simulink model "VehCtrlMdel240818"  (R2018b)
settings: Solver=FixedStepDiscrete  StartTime=0.0  StopTime=10.0  FixedStep=0.0005  RelTol=1e-3  EnableMultiTasking=on
values from neighbouring files (symbols this model uses):
  Ax_OffSet = 0.0    [VehCtrlMdelDictionary.sldd]
  Ay_OffSet = 0.0    [VehCtrlMdelDictionary.sldd]
  Caf = 460.0    [VehCtrlMdelDictionary.sldd]    (also in trqvparameter.m = 460)
  Car = 440.0    [VehCtrlMdelDictionary.sldd]    (also in trqvparameter.m = 440)
  dwf = 1.2    [VehCtrlMdelDictionary.sldd]    (also in trqvparameter.m)
  Iz = 105.0    [VehCtrlMdelDictionary.sldd]    (also in trqvparameter.m = 105)
  Ki = 1.0    [VehCtrlMdelDictionary.sldd]    (also in trqvparameter.m = 20)
  Kp = 2.0    [VehCtrlMdelDictionary.sldd]    (also in trqvparameter.m = 30)
  Ldwf = 1.2    [VehCtrlMdelDictionary.sldd]    (also in trqvparameter.m)
  Ldwr = 1.16    [VehCtrlMdelDictionary.sldd]    (also in trqvparameter.m)
  lf = 0.761    [VehCtrlMdelDictionary.sldd]    (also in trqvparameter.m)
  lr = 0.831    [VehCtrlMdelDictionary.sldd]    (also in trqvparameter.m)
  m = 340.0    [VehCtrlMdelDictionary.sldd]    (also in trqvparameter.m = 340)
  Offset_Angle = 0.0    [VehCtrlMdelDictionary.sldd]
  Qa = 0.1    [VehCtrlMdelDictionary.sldd]    (also in trqvparameter.m)
  Ra = 2.0    [VehCtrlMdelDictionary.sldd]    (also in trqvparameter.m = 2)
  RearRatio = 0.8    [VehCtrlMdelDictionary.sldd]
  Rt = 0.2    [VehCtrlMdelDictionary.sldd]    (also in trqvparameter.m)
  thr1 = 2.0    [VehCtrlMdelDictionary.sldd]    (also in trqvparameter.m = 2)
  thr2 = 0.5    [VehCtrlMdelDictionary.sldd]    (also in trqvparameter.m)
  thr3 = 0.8    [VehCtrlMdelDictionary.sldd]    (also in trqvparameter.m)
  thr4 = 0.5    [VehCtrlMdelDictionary.sldd]    (also in trqvparameter.m)
  thr5 = -0.5    [VehCtrlMdelDictionary.sldd]    (also in trqvparameter.m)
  TrqRquRate = 0.1    [VehCtrlMdelDictionary.sldd]    (also in trqvparameter.m)
  YawRate_OffSet = 0.0    [VehCtrlMdelDictionary.sldd]
undefined symbols (not defined in the file or in its folder): DiscIntNeverNeededParam, I_AN07_5V, I_AN08_5V, I_AN10_5V, I_SW01_L, I_SW02_L, I_SW03_L, O_SW12_HS1A, O_SW14_HS1A, PWM3
libraries: simulink x126, ec5744lib x77, canmsglib x18
(part 5 of 5)

== system VehCtrlMdel240818/Input_Processing/Subsystem/WhlSlpageJudgment/加速度差判断/Filter1 ==
  In : Inport
  Add : Sum
  Constant : Constant  Value=single(-100)
  Constant1 : Constant  Value=single(100)
  Constant2 : Constant  Value=single(100)
  Constant3 : Constant  Value=single(-100)
  Gain : Gain  Gain=0.3
  Gain1 : Gain  Gain=0.7
  Rate Limiter Dynamic : simulink/Discontinuities/Rate Limiter Dynamic
      settings: SourceProductName=Simulink
  Saturation Dynamic : simulink/Discontinuities/Saturation Dynamic  OutMin=[]  OutMax=[]  OutDataTypeStr=Inherit: Same as second input  OutDataType=fixdt(1, 16)  OutScaling=2^-10  DoSatur=off
  Unit Delay : UnitDelay  SampleTime=-1
  Out : Outport  VectorParamsAs1DForOutWhenUnconnected=on
  wires:
  Rate Limiter Dynamic/1 -> Unit Delay/1, Gain1/1
  Gain1/1 -> Add/2
  Add/1 -> Out/1
  Gain/1 -> Add/1
  Unit Delay/1 -> Gain/1
  Constant3/1 -> Rate Limiter Dynamic/3
  Constant2/1 -> Rate Limiter Dynamic/1
  Constant/1 -> Saturation Dynamic/3
  Constant1/1 -> Saturation Dynamic/1
  Saturation Dynamic/1 -> Rate Limiter Dynamic/2
  In/1 -> Saturation Dynamic/2

== system VehCtrlMdel240818/Input_Processing/Subsystem/WhlSlpageJudgment/加速度差判断/Filter2 ==
  In : Inport
  Add : Sum
  Constant : Constant  Value=single(-100)
  Constant1 : Constant  Value=single(100)
  Constant2 : Constant  Value=single(100)
  Constant3 : Constant  Value=single(-100)
  Gain : Gain  Gain=0.3
  Gain1 : Gain  Gain=0.7
  Rate Limiter Dynamic : simulink/Discontinuities/Rate Limiter Dynamic
      settings: SourceProductName=Simulink
  Saturation Dynamic : simulink/Discontinuities/Saturation Dynamic  OutMin=[]  OutMax=[]  OutDataTypeStr=Inherit: Same as second input  OutDataType=fixdt(1, 16)  OutScaling=2^-10  DoSatur=off
  Unit Delay : UnitDelay  SampleTime=-1
  Out : Outport  VectorParamsAs1DForOutWhenUnconnected=on
  wires:
  In/1 -> Saturation Dynamic/2
  Saturation Dynamic/1 -> Rate Limiter Dynamic/2
  Constant1/1 -> Saturation Dynamic/1
  Constant/1 -> Saturation Dynamic/3
  Constant2/1 -> Rate Limiter Dynamic/1
  Constant3/1 -> Rate Limiter Dynamic/3
  Unit Delay/1 -> Gain/1
  Gain/1 -> Add/1
  Add/1 -> Out/1
  Gain1/1 -> Add/2
  Rate Limiter Dynamic/1 -> Gain1/1, Unit Delay/1

== system VehCtrlMdel240818/Input_Processing/Subsystem/WhlSlpageJudgment/加速度差判断/Filter3 ==
  In : Inport
  Add : Sum
  Constant : Constant  Value=single(-100)
  Constant1 : Constant  Value=single(100)
  Constant2 : Constant  Value=single(100)
  Constant3 : Constant  Value=single(-100)
  Gain : Gain  Gain=0.3
  Gain1 : Gain  Gain=0.7
  Rate Limiter Dynamic : simulink/Discontinuities/Rate Limiter Dynamic
      settings: SourceProductName=Simulink
  Saturation Dynamic : simulink/Discontinuities/Saturation Dynamic  OutMin=[]  OutMax=[]  OutDataTypeStr=Inherit: Same as second input  OutDataType=fixdt(1, 16)  OutScaling=2^-10  DoSatur=off
  Unit Delay : UnitDelay  SampleTime=-1
  Out : Outport  VectorParamsAs1DForOutWhenUnconnected=on
  wires:
  Rate Limiter Dynamic/1 -> Unit Delay/1, Gain1/1
  Gain1/1 -> Add/2
  Add/1 -> Out/1
  Gain/1 -> Add/1
  Unit Delay/1 -> Gain/1
  Constant3/1 -> Rate Limiter Dynamic/3
  Constant2/1 -> Rate Limiter Dynamic/1
  Constant/1 -> Saturation Dynamic/3
  Constant1/1 -> Saturation Dynamic/1
  Saturation Dynamic/1 -> Rate Limiter Dynamic/2
  In/1 -> Saturation Dynamic/2

== system VehCtrlMdel240818/Input_Processing/Subsystem/WhlSlpageJudgment/加速度差的微分的判断/Filter ==
  In : Inport
  Add : Sum
  Constant : Constant  Value=single(-100)
  Constant1 : Constant  Value=single(100)
  Constant2 : Constant  Value=single(20)
  Constant3 : Constant  Value=single(-20)
  Gain : Gain  Gain=0.5
  Gain1 : Gain  Gain=0.5
  Rate Limiter Dynamic : simulink/Discontinuities/Rate Limiter Dynamic
      settings: SourceProductName=Simulink
  Saturation Dynamic : simulink/Discontinuities/Saturation Dynamic  OutMin=[]  OutMax=[]  OutDataTypeStr=Inherit: Same as second input  OutDataType=fixdt(1, 16)  OutScaling=2^-10  DoSatur=off
  Unit Delay : UnitDelay  SampleTime=-1
  Out : Outport  VectorParamsAs1DForOutWhenUnconnected=on
  wires:
  In/1 -> Saturation Dynamic/2
  Saturation Dynamic/1 -> Rate Limiter Dynamic/2
  Constant1/1 -> Saturation Dynamic/1
  Constant/1 -> Saturation Dynamic/3
  Constant2/1 -> Rate Limiter Dynamic/1
  Constant3/1 -> Rate Limiter Dynamic/3
  Unit Delay/1 -> Gain/1
  Gain/1 -> Add/1
  Add/1 -> Out/1
  Gain1/1 -> Add/2
  Rate Limiter Dynamic/1 -> Gain1/1, Unit Delay/1

== system VehCtrlMdel240818/Input_Processing/Subsystem/WhlSlpageJudgment/加速度差的微分的判断/Filter1 ==
  In : Inport
  Add : Sum
  Constant : Constant  Value=single(-100)
  Constant1 : Constant  Value=single(100)
  Constant2 : Constant  Value=single(20)
  Constant3 : Constant  Value=single(-20)
  Gain : Gain  Gain=0.5
  Gain1 : Gain  Gain=0.5
  Rate Limiter Dynamic : simulink/Discontinuities/Rate Limiter Dynamic
      settings: SourceProductName=Simulink
  Saturation Dynamic : simulink/Discontinuities/Saturation Dynamic  OutMin=[]  OutMax=[]  OutDataTypeStr=Inherit: Same as second input  OutDataType=fixdt(1, 16)  OutScaling=2^-10  DoSatur=off
  Unit Delay : UnitDelay  SampleTime=-1
  Out : Outport  VectorParamsAs1DForOutWhenUnconnected=on
  wires:
  Rate Limiter Dynamic/1 -> Unit Delay/1, Gain1/1
  Gain1/1 -> Add/2
  Add/1 -> Out/1
  Gain/1 -> Add/1
  Unit Delay/1 -> Gain/1
  Constant3/1 -> Rate Limiter Dynamic/3
  Constant2/1 -> Rate Limiter Dynamic/1
  Constant/1 -> Saturation Dynamic/3
  Constant1/1 -> Saturation Dynamic/1
  Saturation Dynamic/1 -> Rate Limiter Dynamic/2
  In/1 -> Saturation Dynamic/2

== system VehCtrlMdel240818/Input_Processing/Subsystem/WhlSlpageJudgment/加速度差的微分的判断/Filter2 ==
  In : Inport
  Add : Sum
  Constant : Constant  Value=single(-100)
  Constant1 : Constant  Value=single(100)
  Constant2 : Constant  Value=single(20)
  Constant3 : Constant  Value=single(-20)
  Gain : Gain  Gain=0.5
  Gain1 : Gain  Gain=0.5
  Rate Limiter Dynamic : simulink/Discontinuities/Rate Limiter Dynamic
      settings: SourceProductName=Simulink
  Saturation Dynamic : simulink/Discontinuities/Saturation Dynamic  OutMin=[]  OutMax=[]  OutDataTypeStr=Inherit: Same as second input  OutDataType=fixdt(1, 16)  OutScaling=2^-10  DoSatur=off
  Unit Delay : UnitDelay  SampleTime=-1
  Out : Outport  VectorParamsAs1DForOutWhenUnconnected=on
  wires:
  In/1 -> Saturation Dynamic/2
  Saturation Dynamic/1 -> Rate Limiter Dynamic/2
  Constant1/1 -> Saturation Dynamic/1
  Constant/1 -> Saturation Dynamic/3
  Constant2/1 -> Rate Limiter Dynamic/1
  Constant3/1 -> Rate Limiter Dynamic/3
  Unit Delay/1 -> Gain/1
  Gain/1 -> Add/1
  Add/1 -> Out/1
  Gain1/1 -> Add/2
  Rate Limiter Dynamic/1 -> Gain1/1, Unit Delay/1

== system VehCtrlMdel240818/Input_Processing/Subsystem/WhlSlpageJudgment/加速度差的微分的判断/Filter3 ==
  In : Inport
  Add : Sum
  Constant : Constant  Value=single(-100)
  Constant1 : Constant  Value=single(100)
  Constant2 : Constant  Value=single(20)
  Constant3 : Constant  Value=single(-20)
  Gain : Gain  Gain=0.5
  Gain1 : Gain  Gain=0.5
  Rate Limiter Dynamic : simulink/Discontinuities/Rate Limiter Dynamic
      settings: SourceProductName=Simulink
  Saturation Dynamic : simulink/Discontinuities/Saturation Dynamic  OutMin=[]  OutMax=[]  OutDataTypeStr=Inherit: Same as second input  OutDataType=fixdt(1, 16)  OutScaling=2^-10  DoSatur=off
  Unit Delay : UnitDelay  SampleTime=-1
  Out : Outport  VectorParamsAs1DForOutWhenUnconnected=on
  wires:
  Rate Limiter Dynamic/1 -> Unit Delay/1, Gain1/1
  Gain1/1 -> Add/2
  Add/1 -> Out/1
  Gain/1 -> Add/1
  Unit Delay/1 -> Gain/1
  Constant3/1 -> Rate Limiter Dynamic/3
  Constant2/1 -> Rate Limiter Dynamic/1
  Constant/1 -> Saturation Dynamic/3
  Constant1/1 -> Saturation Dynamic/1
  Saturation Dynamic/1 -> Rate Limiter Dynamic/2
  In/1 -> Saturation Dynamic/2

== system VehCtrlMdel240818/Input_Processing/Subsystem/WhlSpdSelect/Subsystem/Subsystem ==
  note: 可在去掉最大最小值里再取最大、最小
  In1 : Inport
  In2 : Inport  Port=2
  In3 : Inport  Port=3
  In4 : Inport  Port=4
  Add : Sum  Commented=on  Inputs=++++
  Add1 : Sum  Commented=on  Inputs=+--
  Add2 : Sum  Commented=on  Inputs=-+
  Compare To Constant1 : simulink/Logic and Bit Operations/Compare To Constant  Commented=on  relop=>  const=0.2  OutDataTypeStr=boolean
  Compare To Constant2 : simulink/Logic and Bit Operations/Compare To Constant  Commented=on  relop=<  const=-0.2  OutDataTypeStr=boolean
  Divide1 : Product  Commented=on  Inputs=*/
  Gain : Gain  Commented=on  Gain=1/2
  Max : MinMax  Commented=on  Function=max  Inputs=3
  Max1 : MinMax  Commented=on  Function=max  Inputs=3
  Max2 : MinMax  Commented=on  Inputs=2
  Max3 : MinMax  Commented=on  Inputs=3
  Max4 : MinMax  Commented=on  Inputs=3
  Max5 : MinMax  Commented=on  Function=max  Inputs=2
  Min1 : MinMax  Commented=on  Function=max  Inputs=4
  Min2 : MinMax  Commented=on  Inputs=4
  NOT : Logic  Commented=on  Operator=NOT  AllPortsSameDT=off  OutDataTypeStr=boolean
  Switch : Switch  Commented=on  Criteria=u2 ~= 0
  Switch1 : Switch  Commented=on  Criteria=u2 ~= 0
  Unit Delay1 : UnitDelay  Commented=on  SampleTime=-1
  steptime1 : Constant  Commented=on  Value=single(0.01)
  Out1 : Outport  VectorParamsAs1DForOutWhenUnconnected=on
  wires:
  Gain/1 -> Switch/3, Unit Delay1/1, Add2/2  "MaxWhlSpd_mps"
  Add2/1 -> Divide1/1
  In1/1 -> Max/1, Max3/1, Add/4, Min1/1, Min2/1
  In4/1 -> Max1/3, Max4/3, Add/1, Min1/4, Min2/4
  In2/1 -> Max/2, Max3/2, Max1/1, Max4/1, Add/3, Min1/2, Min2/2
  In3/1 -> Max/3, Max3/3, Add/2, Min1/3, Min2/3, Max1/2, Max4/2
  Max5/1 -> Switch1/3
  Unit Delay1/1 -> Add2/1
  Max4/1 -> Max5/2
  Compare To Constant2/1 -> Switch/2
  Max3/1 -> Max5/1
  steptime1/1 -> Divide1/2
  Add/1 -> Add1/1
  Compare To Constant1/1 -> NOT/1
  Divide1/1 -> Compare To Constant1/1, Compare To Constant2/1
  Min2/1 -> Add1/2
  Switch1/1 -> Out1/1
  Add1/1 -> Gain/1
  NOT/1 -> Switch1/2
  Max2/1 -> Switch/1
  Max/1 -> Max2/1
  Max1/1 -> Max2/2
  Switch/1 -> Switch1/1
  Min1/1 -> Add1/3

== stateflow chart VehCtrlMdel240818/Drive_Ready/Subsystem/Chart2 ==
  state VehStat [parallel]
    settings: executionOrder=1
    state WaitForEngine
      en:
      send(AMKCANOFF,AMKCANenable);
      send(AMKDCOFF,AMKDCon);
      send(MCDCEnableOFF,MCDCEnable);
      send(InverterOFF,MC_InverterOn);
    state Standby
    state Trans
    state Guard
    state InitStateBack
    state Ready
    state Init
      en:
      errorReset = 1;
    state MCUReadyFail
    WaitForEngine -> Standby : [aMCUReady&&bMCUReady&&cMCUReady]
    Standby -> Guard [order 2] : [KeyPressed&&Brk&&ACC_Release&&cMCUReady&&aMCUReady&&bMCUReady]
    Trans -> Ready : after(2.5,sec){send(EbeepOFF,BeeperStat)}
    Guard -> Trans [order 1] : after(0.25,sec){send(EbeepON,BeeperStat)}
    Guard -> Standby [order 2] : [~KeyPressed||~Brk||~ACC_Release]
    Standby -> WaitForEngine [order 1] : [~aMCUReady||~bMCUReady||~cMCUReady]
    Guard -> InitStateBack [order 3] : [~cMCUReady||~aMCUReady||~bMCUReady]
    Init -> WaitForEngine : [after(1,sec)]
    MCUReadyFail -> WaitForEngine
    InitStateBack -> WaitForEngine
    Ready -> InitStateBack [order 2] : [~HVCutOFF]
    (default) -> Init
    Ready -> MCUReadyFail [order 1] : [~cMCUReady||~aMCUReady||~bMCUReady]
  state BeeperStat [parallel]
    settings: executionOrder=2
    state OFF
    state ON
    (default) -> BeeperStat.OFF
    BeeperStat.OFF -> BeeperStat.ON : EbeepON
    BeeperStat.ON -> BeeperStat.OFF : EbeepOFF
  state AMKDCon [parallel]
    settings: executionOrder=6
    state OFF
    state ON
    (default) -> AMKDCon.OFF
    AMKDCon.OFF -> AMKDCon.ON : AMKDCON
    AMKDCon.ON -> AMKDCon.OFF : AMKDCOFF
  state MCDCEnable [parallel]
    settings: executionOrder=7
    state OFF
    state ON
    (default) -> MCDCEnable.OFF
    MCDCEnable.OFF -> MCDCEnable.ON : MCDCEnableON
    MCDCEnable.ON -> MCDCEnable.OFF : MCDCEnableOFF
  state AMKDCready [parallel]
    settings: executionOrder=4
    state start
    state AMKCAN
      en:
      send(AMKCANON,AMKCANenable);
    state MC_DCready
    state MCDCOncheck
    state DCOnCheckPass
    state MC_DCOnFail
      en:
      send(AMKDCOFF,AMKDCon);
      send(MCDCEnableOFF,MCDCEnable);
      send(InverterOFF,MC_InverterOn);
    state AMKDCOnFinish
    state SYSRDYCECK
    state MCDCEnableState
      en:
      send(MCDCEnableON,MCDCEnable);
    state MC_InverterOn_State
      en:
      send(InverterON,MC_InverterOn);
    (default) -> start
    AMKCAN -> MC_DCready : [SWAMKDCOn]
    MC_DCready -> MCDCOncheck [order 2] : after(0.1,sec){send(AMKDCON,AMKDCon)}
    MCDCOncheck -> DCOnCheckPass [order 1] : after(0.1,sec)
    start -> AMKCAN : after(10,sec)
    DCOnCheckPass -> MCDCEnableState : after(0.1,sec)[MCFLDCOncheck&&MCFRDCOncheck]
    MCDCOncheck -> MC_DCOnFail [order 2] : [~MCFRDCOncheck||~MCFLDCOncheck]
    MC_DCready -> AMKCAN [order 1] : [~SWAMKDCOn]
    SYSRDYCECK -> MC_DCOnFail [order 2] : [~MCFL_SYSREADY||~MCFR_SYSREADY]
    SYSRDYCECK -> AMKDCOnFinish [order 1] : [MCFL_SYSREADY&&MCFR_SYSREADY]
    MC_InverterOn_State -> SYSRDYCECK
    MCDCEnableState -> MC_InverterOn_State : after(0.1,sec)
  state Output [parallel]
    du:
    VehReady = in(VehStat.Ready);
    VehStandby = in(VehStat.Standby);
    BeeperStOut = in(BeeperStat.ON);
    AMKCANready = in(AMKCANenable.ON);
    MCFL_DCOn_setpoints = in(AMKDCon.ON);
    MCFR_DCOn_setpoints = in(AMKDCon.ON);
    MCFL_DCEnable = in(MCDCEnable.ON);
    MCFR_DCEnable = in(MCDCEnable.ON);
    MC_DCOnError = in(AMKDCready.MC_DCOnFail);
    MCFL_InverterOn = in(MC_InverterOn.ON);
    MCFR_InverterOn = in(MC_InverterOn.ON);
    settings: executionOrder=3
  state AMKCANenable [parallel]
    settings: executionOrder=5
    state OFF
    state ON
    (default) -> AMKCANenable.OFF
    AMKCANenable.OFF -> AMKCANenable.ON : AMKCANON
    AMKCANenable.ON -> AMKCANenable.OFF : AMKCANOFF
  state MC_InverterOn [parallel]
    settings: executionOrder=8
    state OFF
    state ON
    (default) -> MC_InverterOn.OFF
    MC_InverterOn.OFF -> MC_InverterOn.ON : InverterON
    MC_InverterOn.ON -> MC_InverterOn.OFF : InverterOFF
  data: Brk input boolean size=1; KeyPressed input boolean size=1; VehReady output boolean size=1; BeeperStOut output boolean size=1; VehStandby output boolean; ACC_Release input boolean; cMCUReady input; aMCUReady input; bMCUReady input; AMKCANready output; MCFL_DCOn_setpoints output; MCFRDCOncheck input; MCFLDCOncheck input; MCFR_DCOn_setpoints output; MCFR_DCEnable output; MCFR_InverterOn output; MC_DCOnError output; MCFL_InverterOn output; MCFL_DCEnable output; MCFL_SYSREADY input; MCFR_SYSREADY input; SWAMKDCOn input; HVCutOFF input; errorReset output
  events: EbeepON local FUNCTION_CALL_EVENT; EbeepOFF local FUNCTION_CALL_EVENT; AMKCANOFF local FUNCTION_CALL_EVENT; AMKCANON local FUNCTION_CALL_EVENT; AMKDCON local FUNCTION_CALL_EVENT; AMKDCOFF local FUNCTION_CALL_EVENT; InverterOFF local FUNCTION_CALL_EVENT; InverterON local FUNCTION_CALL_EVENT; MCDCEnableON local FUNCTION_CALL_EVENT; MCDCEnableOFF local FUNCTION_CALL_EVENT

== matlab function VehCtrlMdel240818/CTRL/MoTrqReq/DYC/Wtarget ==
  data: Vx input size=1; Wtarget output size=1; a input size=1; Car input size=1; Caf input size=1; lr input size=1; lf input size=1; m input; u input; btarget output
function [Wtarget,btarget] = fcn(Vx,a,Car,Caf,lr,lf,m,u)
Wdes = Vx*a/(lf+lr+(m*Vx*Vx*(lr*Car-lf*Caf)/Caf/Car/(lr+lf)/2));
% Wu = 0.85*u*9.8/Vx;
% if abs(Wdes)<=Wu
Wtarget = Wdes;
% else
%    Wtarget = Wu*sign(Wdes);
% end
bdes = (lr-lf*m*Vx*Vx/Car/(lf+lr)/2)*a/(lr+lf+m*Vx*Vx*(lr*Car-lf*Caf)/Car/Caf/(lf+lr)/2);
bu = atan(0.02*u*9.8);
if abs(bdes)<=bu
btarget = bdes;
else
    btarget = bu*sign(bdes);
end

== stateflow chart VehCtrlMdel240818/Input_Processing/Function-Call Subsystem/AccBrkPedal/Timer ==
  state Trigger
    en:
    x = x + 0.01;
    Exit=0;
  state Out
    en:
    Exit=1;
    x=0;
  state InterState
    en:
    x=0;
  Trigger -> Trigger [order 1] : [Trigger&&x<CountTime]
  Trigger -> Out [order 2] : [x>=CountTime]
  (default) -> Trigger
  Out -> Trigger : [~Trigger]
  InterState -> Trigger : [Trigger]
  Trigger -> InterState [order 3] : [x<CountTime&&~Trigger]
  data: Trigger input; CountTime input; Exit output; x local =0

== stateflow chart VehCtrlMdel240818/CTRL/MoTrqReq/DYC/Timer1 ==
  state Trigger
    en:
    x = x + 0.01;
    Exit=0;
  state Out
    en:
    Exit=1;
    x=0;
  state InterState
    en:
    x=0;
  Trigger -> Trigger [order 1] : [Trigger&&x<CountTime]
  Trigger -> Out [order 2] : [x>=CountTime]
  (default) -> Trigger
  Out -> Trigger : [~Trigger]
  InterState -> Trigger : [Trigger]
  Trigger -> InterState [order 3] : [x<CountTime&&~Trigger]
  data: Trigger input; CountTime input; Exit output; x local =0

== stateflow chart VehCtrlMdel240818/CTRL/PwrTrainTempPrtct/Timer1 ==
  state Trigger
    en:
    x = x + 0.01;
    Exit=0;
  state Out
    en:
    Exit=1;
    x=0;
  state InterState
    en:
    x=0;
  Trigger -> Trigger [order 1] : [Trigger&&x<CountTime]
  Trigger -> Out [order 2] : [x>=CountTime]
  (default) -> Trigger
  Out -> Trigger : [~Trigger]
  InterState -> Trigger : [Trigger]
  Trigger -> InterState [order 3] : [x<CountTime&&~Trigger]
  data: Trigger input; CountTime input; Exit output; x local =0

== stateflow chart VehCtrlMdel240818/CTRL/PwrTrainTempPrtct/Timer2 ==
  state Trigger
    en:
    x = x + 0.01;
    Exit=0;
  state Out
    en:
    Exit=1;
    x=0;
  state InterState
    en:
    x=0;
  Trigger -> Trigger [order 1] : [Trigger&&x<CountTime]
  Trigger -> Out [order 2] : [x>=CountTime]
  (default) -> Trigger
  Out -> Trigger : [~Trigger]
  InterState -> Trigger : [Trigger]
  Trigger -> InterState [order 3] : [x<CountTime&&~Trigger]
  data: Trigger input; CountTime input; Exit output; x local =0

== stateflow chart VehCtrlMdel240818/CTRL/MoTrqReq/Chart ==
  state a
  (default) -> a
  data: DYC_Enable input; TCSF_Enable input; TCSR_Enable input; TCSFR_flgActv input; TCSFL_flgActv input; TCSR_flgActv input; TVD_Trigger input; FLModulSW_flag output; FRModulSW_flag output; DYC_Enable1 output; TCSR_Enable1 output; TCSFR_Enable output; TCSFL_Enable output

== stateflow chart VehCtrlMdel240818/Input_Processing/Function-Call Subsystem/SWAS/Timer ==
  state Trigger
    en:
    x = x + 0.01;
    Exit=0;
  state Out
    en:
    Exit=1;
    x=0;
  state InterState
    en:
    x=0;
  Trigger -> Trigger [order 1] : [Trigger&&x<CountTime]
  Trigger -> Out [order 2] : [x>=CountTime]
  (default) -> Trigger
  Out -> Trigger : [~Trigger]
  InterState -> Trigger : [Trigger]
  Trigger -> InterState [order 3] : [x<CountTime&&~Trigger]
  data: Trigger input; CountTime input; Exit output; x local =0

== stateflow chart VehCtrlMdel240818/Input_Processing/Function-Call Subsystem/WhlSpdii_mps/Timer ==
  state Trigger
    en:
    x = x + 0.01;
    Exit=0;
  state Out
    en:
    Exit=1;
    x=0;
  state InterState
    en:
    x=0;
  Trigger -> Trigger [order 1] : [Trigger&&x<CountTime]
  Trigger -> Out [order 2] : [x>=CountTime]
  (default) -> Trigger
  Out -> Trigger : [~Trigger]
  InterState -> Trigger : [Trigger]
  Trigger -> InterState [order 3] : [x<CountTime&&~Trigger]
  data: Trigger input; CountTime input; Exit output; x local =0

== stateflow chart VehCtrlMdel240818/Input_Processing/Function-Call Subsystem/WhlSpdii_mps/Timer1 ==
  state Trigger
    en:
    x = x + 0.01;
    Exit=0;
  state Out
    en:
    Exit=1;
    x=0;
  state InterState
    en:
    x=0;
  Trigger -> Trigger [order 1] : [Trigger&&x<CountTime]
  Trigger -> Out [order 2] : [x>=CountTime]
  (default) -> Trigger
  Out -> Trigger : [~Trigger]
  InterState -> Trigger : [Trigger]
  Trigger -> InterState [order 3] : [x<CountTime&&~Trigger]
  data: Trigger input; CountTime input; Exit output; x local =0

== stateflow chart VehCtrlMdel240818/Input_Processing/Function-Call Subsystem/WhlSpdii_mps/Timer2 ==
  state Trigger
    en:
    x = x + 0.01;
    Exit=0;
  state Out
    en:
    Exit=1;
    x=0;
  state InterState
    en:
    x=0;
  Trigger -> Trigger [order 1] : [Trigger&&x<CountTime]
  Trigger -> Out [order 2] : [x>=CountTime]
  (default) -> Trigger
  Out -> Trigger : [~Trigger]
  InterState -> Trigger : [Trigger]
  Trigger -> InterState [order 3] : [x<CountTime&&~Trigger]
  data: Trigger input; CountTime input; Exit output; x local =0

== stateflow chart VehCtrlMdel240818/Input_Processing/Function-Call Subsystem/WhlSpdii_mps/Timer3 ==
  state Trigger
    en:
    x = x + 0.01;
    Exit=0;
  state Out
    en:
    Exit=1;
    x=0;
  state InterState
    en:
    x=0;
  Trigger -> Trigger [order 1] : [Trigger&&x<CountTime]
  Trigger -> Out [order 2] : [x>=CountTime]
  (default) -> Trigger
  Out -> Trigger : [~Trigger]
  InterState -> Trigger : [Trigger]
  Trigger -> InterState [order 3] : [x<CountTime&&~Trigger]
  data: Trigger input; CountTime input; Exit output; x local =0

== matlab function VehCtrlMdel240818/CTRL/MoTrqReq/DYC/MATLAB Function ==
  data: WSA input; Mz output; WSAV input; lf input; lr input; Caf input; Car input; Iz input; m input; Vx input
function Mz = fcn(WSA,WSAV,lf,lr,Caf,Car,Iz,m,Vx)

Mz = (((lf*lf*Caf+lr*lr*Car)/Iz/Vx)*(-Caf/m/Vx)-((lf*Caf-lr*Car)/m/Vx/Vx-1)*(-lf*Caf/Iz))*Iz*WSA/((lf*Caf-lr*Car)/m/Vx/Vx-1)-(-Caf/m/Vx)*Iz*WSAV/((lf*Caf-lr*Car)/m/Vx/Vx-1);
